simulink model "BatteryFarmTemplate"  (R2022b)
settings: Solver=VariableStepAuto  StartTime=0.0  StopTime=10.0  RelTol=1e-3  AbsTol=1e-3  EnableMultiTasking=on
libraries: ee_lib x242, sdl_lib x84, fl_lib x43
(part 5 of 5)

== system BatteryFarmTemplate/Battery Conex 1/Parallel Charge 6 ==
  Electrical Reference : fl_lib/Electrical/Electrical Elements/Electrical Reference
  Resistor 1 : ee_lib/Passive/Resistor  R=3200 Ohm  enable_R_tol=0  R_tol=5  tol_distribution=1  nSigma=4  enable_operating_limits=0  operating_limit_action=2  max_working_voltage=100 V  power_rating=1 W  enable_faults=0  fault_action=1  R_faulted=inf Ohm  enable_temporal_fault=0  t_fault=1 s  enable_behavioral_fault=0  max_permissible_current=1 A  t_fail_on_current=1 s  noise_mode=0  sample_time=1e-3 s  repeatability=1  auto_seed=4111000739  user_seed=0  Tdevice=25 degC  power_derating_T1=70 degC  power_derating_T2=155 degC  operating_temperature_range_vec=[-50, 150] degC  alpha=3.93e-3 1/K  Tmeas=25 degC  thermal_mass=100 J/K  temperature_specify=off  temperature_priority=High  temperature=298.15 K  temperature_nominal_specify=off  temperature_nominal_unit=K  temperature_nominal_value=1
  Resistor 2 : ee_lib/Passive/Resistor  R=450 Ohm  enable_R_tol=0  R_tol=5  tol_distribution=1  nSigma=4  enable_operating_limits=0  operating_limit_action=2  max_working_voltage=100 V  power_rating=1 W  enable_faults=0  fault_action=1  R_faulted=inf Ohm  enable_temporal_fault=0  t_fault=1 s  enable_behavioral_fault=0  max_permissible_current=1 A  t_fail_on_current=1 s  noise_mode=0  sample_time=1e-3 s  repeatability=1  auto_seed=2084672538  user_seed=0  Tdevice=25 degC  power_derating_T1=70 degC  power_derating_T2=155 degC  operating_temperature_range_vec=[-50, 150] degC  alpha=3.93e-3 1/K  Tmeas=25 degC  thermal_mass=100 J/K  temperature_specify=off  temperature_priority=High  temperature=298.15 K  temperature_nominal_specify=off  temperature_nominal_unit=K  temperature_nominal_value=1
  SPST Relay 1 : ee_lib/Switches & Breakers/Relays/SPST Relay  block_choices=ee.enum.controlport.ps  R_closed=0.01 Ohm  G_open=1e-8 1/Ohm  Threshold=0  exposemeasurement=ee.enum.exposemeasurement.hidden  V_rated=5 V  V_energize=75  V_deenergize=25  l_winding=0.08 H  r_winding=12.5 Ohm  g_winding=1e-9 1/Ohm  T_brk_C_S=0 s  T_mak_C_S=0 s  enable_faults=ee.enum.relays.enable.no  fault_action=ee.enum.relays.faultaction.none  fault_types=ee.enum.relays.faultTypes.winding  fault_condition_ps=ee.enum.relays.faultConditionSPSTps.csstuck  r_deg_closed_s=1e-9 Ohm  winding_tau_fault=1e-3 s  tau_fault=1e-3 s  enable_temporal_fault=ee.enum.relays.enable.no  t_fault_stick=1 s  t_fault_ComOpen=1 s  t_fault=1 s  enable_behavioral_fault=ee.enum.relays.enable.no  winding_max_permissible_voltage=inf V  n_fail_on_voltage=1  winding_max_permissible_current=inf A  max_permissible_current=inf A  t_fail_on_current=1 s
      settings: InternalSimscapePortConfiguration="{\"Bottom\":[],\"Left\":[{\"id\":\"PS\",\"label\":\"PS\",\"type\":\"input\"}],\"Right\":[{\"id\":\"S\",\"label\":\"S\",\"type\":\"foundation.electrical.electrical\"},{\"id\":\"COM\",\"label\":\"C\",\"type\":\"foundation.electrical.electrical\"}],\"Top\":[]}"
  SPST Relay 2 : ee_lib/Switches & Breakers/Relays/SPST Relay  block_choices=ee.enum.controlport.ps  R_closed=0.01 Ohm  G_open=1e-8 1/Ohm  Threshold=0  exposemeasurement=ee.enum.exposemeasurement.hidden  V_rated=5 V  V_energize=75  V_deenergize=25  l_winding=0.08 H  r_winding=12.5 Ohm  g_winding=1e-9 1/Ohm  T_brk_C_S=0 s  T_mak_C_S=0 s  enable_faults=ee.enum.relays.enable.no  fault_action=ee.enum.relays.faultaction.none  fault_types=ee.enum.relays.faultTypes.winding  fault_condition_ps=ee.enum.relays.faultConditionSPSTps.csstuck  r_deg_closed_s=1e-9 Ohm  winding_tau_fault=1e-3 s  tau_fault=1e-3 s  enable_temporal_fault=ee.enum.relays.enable.no  t_fault_stick=1 s  t_fault_ComOpen=1 s  t_fault=1 s  enable_behavioral_fault=ee.enum.relays.enable.no  winding_max_permissible_voltage=inf V  n_fail_on_voltage=1  winding_max_permissible_current=inf A  max_permissible_current=inf A  t_fail_on_current=1 s
      settings: InternalSimscapePortConfiguration="{\"Bottom\":[],\"Left\":[{\"id\":\"PS\",\"label\":\"PS\",\"type\":\"input\"}],\"Right\":[{\"id\":\"S\",\"label\":\"S\",\"type\":\"foundation.electrical.electrical\"},{\"id\":\"COM\",\"label\":\"C\",\"type\":\"foundation.electrical.electrical\"}],\"Top\":[]}"
  Charge Pos In : PMIOPort  Side=Left
  Charge Pos Out : PMIOPort  Port=2  Side=Left
  Energize Relay : PMIOPort  Port=3  Side=Left
  Charge Neg Out : PMIOPort  Port=4  Side=Right
  Charge Neg In : PMIOPort  Port=5  Side=Right
  connections:
  Electrical Reference/LConn1 -- Resistor 2/RConn1
  Resistor 2/LConn1 -- Resistor 1/LConn1 -- SPST Relay 1/RConn1
  SPST Relay 2/RConn2 -- Charge Neg Out/RConn1
  Charge Neg In/RConn1 -- SPST Relay 2/RConn1
  Resistor 1/RConn1 -- Charge Pos In/RConn1
  Charge Pos Out/RConn1 -- SPST Relay 1/RConn2
  SPST Relay 1/LConn1 -- Energize Relay/RConn1 -- SPST Relay 2/LConn1

== system BatteryFarmTemplate/Battery Conex 1/Parallel Charge 7 ==
  Electrical Reference : fl_lib/Electrical/Electrical Elements/Electrical Reference
  Resistor 1 : ee_lib/Passive/Resistor  R=3200 Ohm  enable_R_tol=0  R_tol=5  tol_distribution=1  nSigma=4  enable_operating_limits=0  operating_limit_action=2  max_working_voltage=100 V  power_rating=1 W  enable_faults=0  fault_action=1  R_faulted=inf Ohm  enable_temporal_fault=0  t_fault=1 s  enable_behavioral_fault=0  max_permissible_current=1 A  t_fail_on_current=1 s  noise_mode=0  sample_time=1e-3 s  repeatability=1  auto_seed=3437178441  user_seed=0  Tdevice=25 degC  power_derating_T1=70 degC  power_derating_T2=155 degC  operating_temperature_range_vec=[-50, 150] degC  alpha=3.93e-3 1/K  Tmeas=25 degC  thermal_mass=100 J/K  temperature_specify=off  temperature_priority=High  temperature=298.15 K  temperature_nominal_specify=off  temperature_nominal_unit=K  temperature_nominal_value=1
  Resistor 2 : ee_lib/Passive/Resistor  R=450 Ohm  enable_R_tol=0  R_tol=5  tol_distribution=1  nSigma=4  enable_operating_limits=0  operating_limit_action=2  max_working_voltage=100 V  power_rating=1 W  enable_faults=0  fault_action=1  R_faulted=inf Ohm  enable_temporal_fault=0  t_fault=1 s  enable_behavioral_fault=0  max_permissible_current=1 A  t_fail_on_current=1 s  noise_mode=0  sample_time=1e-3 s  repeatability=1  auto_seed=609397185  user_seed=0  Tdevice=25 degC  power_derating_T1=70 degC  power_derating_T2=155 degC  operating_temperature_range_vec=[-50, 150] degC  alpha=3.93e-3 1/K  Tmeas=25 degC  thermal_mass=100 J/K  temperature_specify=off  temperature_priority=High  temperature=298.15 K  temperature_nominal_specify=off  temperature_nominal_unit=K  temperature_nominal_value=1
  SPST Relay 1 : ee_lib/Switches & Breakers/Relays/SPST Relay  block_choices=ee.enum.controlport.ps  R_closed=0.01 Ohm  G_open=1e-8 1/Ohm  Threshold=0  exposemeasurement=ee.enum.exposemeasurement.hidden  V_rated=5 V  V_energize=75  V_deenergize=25  l_winding=0.08 H  r_winding=12.5 Ohm  g_winding=1e-9 1/Ohm  T_brk_C_S=0 s  T_mak_C_S=0 s  enable_faults=ee.enum.relays.enable.no  fault_action=ee.enum.relays.faultaction.none  fault_types=ee.enum.relays.faultTypes.winding  fault_condition_ps=ee.enum.relays.faultConditionSPSTps.csstuck  r_deg_closed_s=1e-9 Ohm  winding_tau_fault=1e-3 s  tau_fault=1e-3 s  enable_temporal_fault=ee.enum.relays.enable.no  t_fault_stick=1 s  t_fault_ComOpen=1 s  t_fault=1 s  enable_behavioral_fault=ee.enum.relays.enable.no  winding_max_permissible_voltage=inf V  n_fail_on_voltage=1  winding_max_permissible_current=inf A  max_permissible_current=inf A  t_fail_on_current=1 s
      settings: InternalSimscapePortConfiguration="{\"Bottom\":[],\"Left\":[{\"id\":\"PS\",\"label\":\"PS\",\"type\":\"input\"}],\"Right\":[{\"id\":\"S\",\"label\":\"S\",\"type\":\"foundation.electrical.electrical\"},{\"id\":\"COM\",\"label\":\"C\",\"type\":\"foundation.electrical.electrical\"}],\"Top\":[]}"
  SPST Relay 2 : ee_lib/Switches & Breakers/Relays/SPST Relay  block_choices=ee.enum.controlport.ps  R_closed=0.01 Ohm  G_open=1e-8 1/Ohm  Threshold=0  exposemeasurement=ee.enum.exposemeasurement.hidden  V_rated=5 V  V_energize=75  V_deenergize=25  l_winding=0.08 H  r_winding=12.5 Ohm  g_winding=1e-9 1/Ohm  T_brk_C_S=0 s  T_mak_C_S=0 s  enable_faults=ee.enum.relays.enable.no  fault_action=ee.enum.relays.faultaction.none  fault_types=ee.enum.relays.faultTypes.winding  fault_condition_ps=ee.enum.relays.faultConditionSPSTps.csstuck  r_deg_closed_s=1e-9 Ohm  winding_tau_fault=1e-3 s  tau_fault=1e-3 s  enable_temporal_fault=ee.enum.relays.enable.no  t_fault_stick=1 s  t_fault_ComOpen=1 s  t_fault=1 s  enable_behavioral_fault=ee.enum.relays.enable.no  winding_max_permissible_voltage=inf V  n_fail_on_voltage=1  winding_max_permissible_current=inf A  max_permissible_current=inf A  t_fail_on_current=1 s
      settings: InternalSimscapePortConfiguration="{\"Bottom\":[],\"Left\":[{\"id\":\"PS\",\"label\":\"PS\",\"type\":\"input\"}],\"Right\":[{\"id\":\"S\",\"label\":\"S\",\"type\":\"foundation.electrical.electrical\"},{\"id\":\"COM\",\"label\":\"C\",\"type\":\"foundation.electrical.electrical\"}],\"Top\":[]}"
  Charge Pos In : PMIOPort  Side=Left
  Charge Pos Out : PMIOPort  Port=2  Side=Left
  Energize Relay : PMIOPort  Port=3  Side=Left
  Charge Neg Out : PMIOPort  Port=4  Side=Right
  Charge Neg In : PMIOPort  Port=5  Side=Right
  connections:
  Electrical Reference/LConn1 -- Resistor 2/RConn1
  Resistor 2/LConn1 -- Resistor 1/LConn1 -- SPST Relay 1/RConn1
  SPST Relay 2/RConn2 -- Charge Neg Out/RConn1
  Charge Neg In/RConn1 -- SPST Relay 2/RConn1
  Resistor 1/RConn1 -- Charge Pos In/RConn1
  Charge Pos Out/RConn1 -- SPST Relay 1/RConn2
  SPST Relay 1/LConn1 -- Energize Relay/RConn1 -- SPST Relay 2/LConn1

== system BatteryFarmTemplate/Battery Conex 1/Parallel Charge 8 ==
  Electrical Reference : fl_lib/Electrical/Electrical Elements/Electrical Reference
  Resistor 1 : ee_lib/Passive/Resistor  R=3200 Ohm  enable_R_tol=0  R_tol=5  tol_distribution=1  nSigma=4  enable_operating_limits=0  operating_limit_action=2  max_working_voltage=100 V  power_rating=1 W  enable_faults=0  fault_action=1  R_faulted=inf Ohm  enable_temporal_fault=0  t_fault=1 s  enable_behavioral_fault=0  max_permissible_current=1 A  t_fail_on_current=1 s  noise_mode=0  sample_time=1e-3 s  repeatability=1  auto_seed=802611725  user_seed=0  Tdevice=25 degC  power_derating_T1=70 degC  power_derating_T2=155 degC  operating_temperature_range_vec=[-50, 150] degC  alpha=3.93e-3 1/K  Tmeas=25 degC  thermal_mass=100 J/K  temperature_specify=off  temperature_priority=High  temperature=298.15 K  temperature_nominal_specify=off  temperature_nominal_unit=K  temperature_nominal_value=1
  Resistor 2 : ee_lib/Passive/Resistor  R=450 Ohm  enable_R_tol=0  R_tol=5  tol_distribution=1  nSigma=4  enable_operating_limits=0  operating_limit_action=2  max_working_voltage=100 V  power_rating=1 W  enable_faults=0  fault_action=1  R_faulted=inf Ohm  enable_temporal_fault=0  t_fault=1 s  enable_behavioral_fault=0  max_permissible_current=1 A  t_fail_on_current=1 s  noise_mode=0  sample_time=1e-3 s  repeatability=1  auto_seed=2103522063  user_seed=0  Tdevice=25 degC  power_derating_T1=70 degC  power_derating_T2=155 degC  operating_temperature_range_vec=[-50, 150] degC  alpha=3.93e-3 1/K  Tmeas=25 degC  thermal_mass=100 J/K  temperature_specify=off  temperature_priority=High  temperature=298.15 K  temperature_nominal_specify=off  temperature_nominal_unit=K  temperature_nominal_value=1
  SPST Relay 1 : ee_lib/Switches & Breakers/Relays/SPST Relay  block_choices=ee.enum.controlport.ps  R_closed=0.01 Ohm  G_open=1e-8 1/Ohm  Threshold=0  exposemeasurement=ee.enum.exposemeasurement.hidden  V_rated=5 V  V_energize=75  V_deenergize=25  l_winding=0.08 H  r_winding=12.5 Ohm  g_winding=1e-9 1/Ohm  T_brk_C_S=0 s  T_mak_C_S=0 s  enable_faults=ee.enum.relays.enable.no  fault_action=ee.enum.relays.faultaction.none  fault_types=ee.enum.relays.faultTypes.winding  fault_condition_ps=ee.enum.relays.faultConditionSPSTps.csstuck  r_deg_closed_s=1e-9 Ohm  winding_tau_fault=1e-3 s  tau_fault=1e-3 s  enable_temporal_fault=ee.enum.relays.enable.no  t_fault_stick=1 s  t_fault_ComOpen=1 s  t_fault=1 s  enable_behavioral_fault=ee.enum.relays.enable.no  winding_max_permissible_voltage=inf V  n_fail_on_voltage=1  winding_max_permissible_current=inf A  max_permissible_current=inf A  t_fail_on_current=1 s
      settings: InternalSimscapePortConfiguration="{\"Bottom\":[],\"Left\":[{\"id\":\"PS\",\"label\":\"PS\",\"type\":\"input\"}],\"Right\":[{\"id\":\"S\",\"label\":\"S\",\"type\":\"foundation.electrical.electrical\"},{\"id\":\"COM\",\"label\":\"C\",\"type\":\"foundation.electrical.electrical\"}],\"Top\":[]}"
  SPST Relay 2 : ee_lib/Switches & Breakers/Relays/SPST Relay  block_choices=ee.enum.controlport.ps  R_closed=0.01 Ohm  G_open=1e-8 1/Ohm  Threshold=0  exposemeasurement=ee.enum.exposemeasurement.hidden  V_rated=5 V  V_energize=75  V_deenergize=25  l_winding=0.08 H  r_winding=12.5 Ohm  g_winding=1e-9 1/Ohm  T_brk_C_S=0 s  T_mak_C_S=0 s  enable_faults=ee.enum.relays.enable.no  fault_action=ee.enum.relays.faultaction.none  fault_types=ee.enum.relays.faultTypes.winding  fault_condition_ps=ee.enum.relays.faultConditionSPSTps.csstuck  r_deg_closed_s=1e-9 Ohm  winding_tau_fault=1e-3 s  tau_fault=1e-3 s  enable_temporal_fault=ee.enum.relays.enable.no  t_fault_stick=1 s  t_fault_ComOpen=1 s  t_fault=1 s  enable_behavioral_fault=ee.enum.relays.enable.no  winding_max_permissible_voltage=inf V  n_fail_on_voltage=1  winding_max_permissible_current=inf A  max_permissible_current=inf A  t_fail_on_current=1 s
      settings: InternalSimscapePortConfiguration="{\"Bottom\":[],\"Left\":[{\"id\":\"PS\",\"label\":\"PS\",\"type\":\"input\"}],\"Right\":[{\"id\":\"S\",\"label\":\"S\",\"type\":\"foundation.electrical.electrical\"},{\"id\":\"COM\",\"label\":\"C\",\"type\":\"foundation.electrical.electrical\"}],\"Top\":[]}"
  Charge Pos In : PMIOPort  Side=Left
  Charge Pos Out : PMIOPort  Port=2  Side=Left
  Energize Relay : PMIOPort  Port=3  Side=Left
  Charge Neg Out : PMIOPort  Port=4  Side=Right
  Charge Neg In : PMIOPort  Port=5  Side=Right
  connections:
  Electrical Reference/LConn1 -- Resistor 2/RConn1
  Resistor 2/LConn1 -- Resistor 1/LConn1 -- SPST Relay 1/RConn1
  SPST Relay 2/RConn2 -- Charge Neg Out/RConn1
  Charge Neg In/RConn1 -- SPST Relay 2/RConn1
  Resistor 1/RConn1 -- Charge Pos In/RConn1
  Charge Pos Out/RConn1 -- SPST Relay 1/RConn2
  SPST Relay 1/LConn1 -- Energize Relay/RConn1 -- SPST Relay 2/LConn1

== system BatteryFarmTemplate/Battery Conex 1/Parallel Charge 9 ==
  Electrical Reference : fl_lib/Electrical/Electrical Elements/Electrical Reference
  Resistor 1 : ee_lib/Passive/Resistor  R=3200 Ohm  enable_R_tol=0  R_tol=5  tol_distribution=1  nSigma=4  enable_operating_limits=0  operating_limit_action=2  max_working_voltage=100 V  power_rating=1 W  enable_faults=0  fault_action=1  R_faulted=inf Ohm  enable_temporal_fault=0  t_fault=1 s  enable_behavioral_fault=0  max_permissible_current=1 A  t_fail_on_current=1 s  noise_mode=0  sample_time=1e-3 s  repeatability=1  auto_seed=1913778160  user_seed=0  Tdevice=25 degC  power_derating_T1=70 degC  power_derating_T2=155 degC  operating_temperature_range_vec=[-50, 150] degC  alpha=3.93e-3 1/K  Tmeas=25 degC  thermal_mass=100 J/K  temperature_specify=off  temperature_priority=High  temperature=298.15 K  temperature_nominal_specify=off  temperature_nominal_unit=K  temperature_nominal_value=1
  Resistor 2 : ee_lib/Passive/Resistor  R=450 Ohm  enable_R_tol=0  R_tol=5  tol_distribution=1  nSigma=4  enable_operating_limits=0  operating_limit_action=2  max_working_voltage=100 V  power_rating=1 W  enable_faults=0  fault_action=1  R_faulted=inf Ohm  enable_temporal_fault=0  t_fault=1 s  enable_behavioral_fault=0  max_permissible_current=1 A  t_fail_on_current=1 s  noise_mode=0  sample_time=1e-3 s  repeatability=1  auto_seed=2775893241  user_seed=0  Tdevice=25 degC  power_derating_T1=70 degC  power_derating_T2=155 degC  operating_temperature_range_vec=[-50, 150] degC  alpha=3.93e-3 1/K  Tmeas=25 degC  thermal_mass=100 J/K  temperature_specify=off  temperature_priority=High  temperature=298.15 K  temperature_nominal_specify=off  temperature_nominal_unit=K  temperature_nominal_value=1
  SPST Relay 1 : ee_lib/Switches & Breakers/Relays/SPST Relay  block_choices=ee.enum.controlport.ps  R_closed=0.01 Ohm  G_open=1e-8 1/Ohm  Threshold=0  exposemeasurement=ee.enum.exposemeasurement.hidden  V_rated=5 V  V_energize=75  V_deenergize=25  l_winding=0.08 H  r_winding=12.5 Ohm  g_winding=1e-9 1/Ohm  T_brk_C_S=0 s  T_mak_C_S=0 s  enable_faults=ee.enum.relays.enable.no  fault_action=ee.enum.relays.faultaction.none  fault_types=ee.enum.relays.faultTypes.winding  fault_condition_ps=ee.enum.relays.faultConditionSPSTps.csstuck  r_deg_closed_s=1e-9 Ohm  winding_tau_fault=1e-3 s  tau_fault=1e-3 s  enable_temporal_fault=ee.enum.relays.enable.no  t_fault_stick=1 s  t_fault_ComOpen=1 s  t_fault=1 s  enable_behavioral_fault=ee.enum.relays.enable.no  winding_max_permissible_voltage=inf V  n_fail_on_voltage=1  winding_max_permissible_current=inf A  max_permissible_current=inf A  t_fail_on_current=1 s
      settings: InternalSimscapePortConfiguration="{\"Bottom\":[],\"Left\":[{\"id\":\"PS\",\"label\":\"PS\",\"type\":\"input\"}],\"Right\":[{\"id\":\"S\",\"label\":\"S\",\"type\":\"foundation.electrical.electrical\"},{\"id\":\"COM\",\"label\":\"C\",\"type\":\"foundation.electrical.electrical\"}],\"Top\":[]}"
  SPST Relay 2 : ee_lib/Switches & Breakers/Relays/SPST Relay  block_choices=ee.enum.controlport.ps  R_closed=0.01 Ohm  G_open=1e-8 1/Ohm  Threshold=0  exposemeasurement=ee.enum.exposemeasurement.hidden  V_rated=5 V  V_energize=75  V_deenergize=25  l_winding=0.08 H  r_winding=12.5 Ohm  g_winding=1e-9 1/Ohm  T_brk_C_S=0 s  T_mak_C_S=0 s  enable_faults=ee.enum.relays.enable.no  fault_action=ee.enum.relays.faultaction.none  fault_types=ee.enum.relays.faultTypes.winding  fault_condition_ps=ee.enum.relays.faultConditionSPSTps.csstuck  r_deg_closed_s=1e-9 Ohm  winding_tau_fault=1e-3 s  tau_fault=1e-3 s  enable_temporal_fault=ee.enum.relays.enable.no  t_fault_stick=1 s  t_fault_ComOpen=1 s  t_fault=1 s  enable_behavioral_fault=ee.enum.relays.enable.no  winding_max_permissible_voltage=inf V  n_fail_on_voltage=1  winding_max_permissible_current=inf A  max_permissible_current=inf A  t_fail_on_current=1 s
      settings: InternalSimscapePortConfiguration="{\"Bottom\":[],\"Left\":[{\"id\":\"PS\",\"label\":\"PS\",\"type\":\"input\"}],\"Right\":[{\"id\":\"S\",\"label\":\"S\",\"type\":\"foundation.electrical.electrical\"},{\"id\":\"COM\",\"label\":\"C\",\"type\":\"foundation.electrical.electrical\"}],\"Top\":[]}"
  Charge Pos In : PMIOPort  Side=Left
  Charge Pos Out : PMIOPort  Port=2  Side=Left
  Energize Relay : PMIOPort  Port=3  Side=Left
  Charge Neg Out : PMIOPort  Port=4  Side=Right
  Charge Neg In : PMIOPort  Port=5  Side=Right
  connections:
  Electrical Reference/LConn1 -- Resistor 2/RConn1
  Resistor 2/LConn1 -- Resistor 1/LConn1 -- SPST Relay 1/RConn1
  SPST Relay 2/RConn2 -- Charge Neg Out/RConn1
  Charge Neg In/RConn1 -- SPST Relay 2/RConn1
  Resistor 1/RConn1 -- Charge Pos In/RConn1
  Charge Pos Out/RConn1 -- SPST Relay 1/RConn2
  SPST Relay 1/LConn1 -- Energize Relay/RConn1 -- SPST Relay 2/LConn1

== system BatteryFarmTemplate/Battery Conex 1/Parallel Relay Control ==
  Parallel 1 : PMIOPort  Side=Right
  Parallel 2 : PMIOPort  Port=2  Side=Right
  Parallel 3 : PMIOPort  Port=3  Side=Right
  Parallel 4 : PMIOPort  Port=4  Side=Right
  Parallel 5 : PMIOPort  Port=5  Side=Right
  Parallel 6 : PMIOPort  Port=6  Side=Right
  Parallel 7 : PMIOPort  Port=7  Side=Right
  Parallel 8 : PMIOPort  Port=8  Side=Right
  Parallel 9 : PMIOPort  Port=9  Side=Right
  Parallel 10 : PMIOPort  Port=10  Side=Right
  Parallel 11 : PMIOPort  Port=11  Side=Right
  Parallel 12 : PMIOPort  Port=12  Side=Right
  Parallel 13 : PMIOPort  Port=13  Side=Right
  Parallel 14 : PMIOPort  Port=14  Side=Right

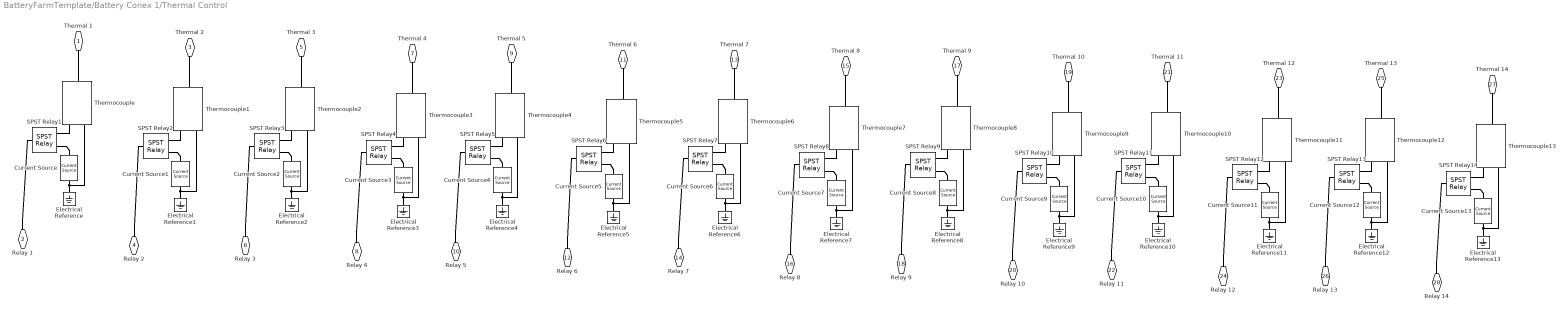
== system BatteryFarmTemplate/Battery Conex 1/Thermal Control ==
  Current Source : ee_lib/Sources/Current Source  dc_current=44 A  ac_current=0 A  ac_shift=0 rad  ac_frequency=50 Hz  noise_mode=ee.enum.sources.noise.Disabled  PSD=0 A^2/Hz  sample_time=1e-3 s  repeatability=ee.enum.sources.repeatability.NotRepeatable  user_seed=0  auto_seed=3890346746  i_specify=off  i_priority=None  i=0 A  i_nominal_specify=off  i_nominal_unit=A  i_nominal_value=1  v_specify=off  v_priority=None  v=0 V  v_nominal_specify=off  v_nominal_unit=V  v_nominal_value=1
  Current Source1 : ee_lib/Sources/Current Source  dc_current=44 A  ac_current=0 A  ac_shift=0 rad  ac_frequency=50 Hz  noise_mode=ee.enum.sources.noise.Disabled  PSD=0 A^2/Hz  sample_time=1e-3 s  repeatability=ee.enum.sources.repeatability.NotRepeatable  user_seed=0  auto_seed=609397185  i_specify=off  i_priority=None  i=0 A  i_nominal_specify=off  i_nominal_unit=A  i_nominal_value=1  v_specify=off  v_priority=None  v=0 V  v_nominal_specify=off  v_nominal_unit=V  v_nominal_value=1
  Current Source10 : ee_lib/Sources/Current Source  dc_current=44 A  ac_current=0 A  ac_shift=0 rad  ac_frequency=50 Hz  noise_mode=ee.enum.sources.noise.Disabled  PSD=0 A^2/Hz  sample_time=1e-3 s  repeatability=ee.enum.sources.repeatability.NotRepeatable  user_seed=0  auto_seed=2816384857  i_specify=off  i_priority=None  i=0 A  i_nominal_specify=off  i_nominal_unit=A  i_nominal_value=1  v_specify=off  v_priority=None  v=0 V  v_nominal_specify=off  v_nominal_unit=V  v_nominal_value=1
  Current Source11 : ee_lib/Sources/Current Source  dc_current=44 A  ac_current=0 A  ac_shift=0 rad  ac_frequency=50 Hz  noise_mode=ee.enum.sources.noise.Disabled  PSD=0 A^2/Hz  sample_time=1e-3 s  repeatability=ee.enum.sources.repeatability.NotRepeatable  user_seed=0  auto_seed=153380492  i_specify=off  i_priority=None  i=0 A  i_nominal_specify=off  i_nominal_unit=A  i_nominal_value=1  v_specify=off  v_priority=None  v=0 V  v_nominal_specify=off  v_nominal_unit=V  v_nominal_value=1
  Current Source12 : ee_lib/Sources/Current Source  dc_current=44 A  ac_current=0 A  ac_shift=0 rad  ac_frequency=50 Hz  noise_mode=ee.enum.sources.noise.Disabled  PSD=0 A^2/Hz  sample_time=1e-3 s  repeatability=ee.enum.sources.repeatability.NotRepeatable  user_seed=0  auto_seed=3191729647  i_specify=off  i_priority=None  i=0 A  i_nominal_specify=off  i_nominal_unit=A  i_nominal_value=1  v_specify=off  v_priority=None  v=0 V  v_nominal_specify=off  v_nominal_unit=V  v_nominal_value=1
  Current Source13 : ee_lib/Sources/Current Source  dc_current=44 A  ac_current=0 A  ac_shift=0 rad  ac_frequency=50 Hz  noise_mode=ee.enum.sources.noise.Disabled  PSD=0 A^2/Hz  sample_time=1e-3 s  repeatability=ee.enum.sources.repeatability.NotRepeatable  user_seed=0  auto_seed=1684602222  i_specify=off  i_priority=None  i=0 A  i_nominal_specify=off  i_nominal_unit=A  i_nominal_value=1  v_specify=off  v_priority=None  v=0 V  v_nominal_specify=off  v_nominal_unit=V  v_nominal_value=1
  Current Source2 : ee_lib/Sources/Current Source  dc_current=44 A  ac_current=0 A  ac_shift=0 rad  ac_frequency=50 Hz  noise_mode=ee.enum.sources.noise.Disabled  PSD=0 A^2/Hz  sample_time=1e-3 s  repeatability=ee.enum.sources.repeatability.NotRepeatable  user_seed=0  auto_seed=1811450916  i_specify=off  i_priority=None  i=0 A  i_nominal_specify=off  i_nominal_unit=A  i_nominal_value=1  v_specify=off  v_priority=None  v=0 V  v_nominal_specify=off  v_nominal_unit=V  v_nominal_value=1
  Current Source3 : ee_lib/Sources/Current Source  dc_current=44 A  ac_current=0 A  ac_shift=0 rad  ac_frequency=50 Hz  noise_mode=ee.enum.sources.noise.Disabled  PSD=0 A^2/Hz  sample_time=1e-3 s  repeatability=ee.enum.sources.repeatability.NotRepeatable  user_seed=0  auto_seed=3933054132  i_specify=off  i_priority=None  i=0 A  i_nominal_specify=off  i_nominal_unit=A  i_nominal_value=1  v_specify=off  v_priority=None  v=0 V  v_nominal_specify=off  v_nominal_unit=V  v_nominal_value=1
  Current Source4 : ee_lib/Sources/Current Source  dc_current=44 A  ac_current=0 A  ac_shift=0 rad  ac_frequency=50 Hz  noise_mode=ee.enum.sources.noise.Disabled  PSD=0 A^2/Hz  sample_time=1e-3 s  repeatability=ee.enum.sources.repeatability.NotRepeatable  user_seed=0  auto_seed=3402504572  i_specify=off  i_priority=None  i=0 A  i_nominal_specify=off  i_nominal_unit=A  i_nominal_value=1  v_specify=off  v_priority=None  v=0 V  v_nominal_specify=off  v_nominal_unit=V  v_nominal_value=1
  Current Source5 : ee_lib/Sources/Current Source  dc_current=44 A  ac_current=0 A  ac_shift=0 rad  ac_frequency=50 Hz  noise_mode=ee.enum.sources.noise.Disabled  PSD=0 A^2/Hz  sample_time=1e-3 s  repeatability=ee.enum.sources.repeatability.NotRepeatable  user_seed=0  auto_seed=4120988592  i_specify=off  i_priority=None  i=0 A  i_nominal_specify=off  i_nominal_unit=A  i_nominal_value=1  v_specify=off  v_priority=None  v=0 V  v_nominal_specify=off  v_nominal_unit=V  v_nominal_value=1
  Current Source6 : ee_lib/Sources/Current Source  dc_current=44 A  ac_current=0 A  ac_shift=0 rad  ac_frequency=50 Hz  noise_mode=ee.enum.sources.noise.Disabled  PSD=0 A^2/Hz  sample_time=1e-3 s  repeatability=ee.enum.sources.repeatability.NotRepeatable  user_seed=0  auto_seed=3646982598  i_specify=off  i_priority=None  i=0 A  i_nominal_specify=off  i_nominal_unit=A  i_nominal_value=1  v_specify=off  v_priority=None  v=0 V  v_nominal_specify=off  v_nominal_unit=V  v_nominal_value=1
  Current Source7 : ee_lib/Sources/Current Source  dc_current=44 A  ac_current=0 A  ac_shift=0 rad  ac_frequency=50 Hz  noise_mode=ee.enum.sources.noise.Disabled  PSD=0 A^2/Hz  sample_time=1e-3 s  repeatability=ee.enum.sources.repeatability.NotRepeatable  user_seed=0  auto_seed=4011470453  i_specify=off  i_priority=None  i=0 A  i_nominal_specify=off  i_nominal_unit=A  i_nominal_value=1  v_specify=off  v_priority=None  v=0 V  v_nominal_specify=off  v_nominal_unit=V  v_nominal_value=1
  Current Source8 : ee_lib/Sources/Current Source  dc_current=44 A  ac_current=0 A  ac_shift=0 rad  ac_frequency=50 Hz  noise_mode=ee.enum.sources.noise.Disabled  PSD=0 A^2/Hz  sample_time=1e-3 s  repeatability=ee.enum.sources.repeatability.NotRepeatable  user_seed=0  auto_seed=2915145293  i_specify=off  i_priority=None  i=0 A  i_nominal_specify=off  i_nominal_unit=A  i_nominal_value=1  v_specify=off  v_priority=None  v=0 V  v_nominal_specify=off  v_nominal_unit=V  v_nominal_value=1
  Current Source9 : ee_lib/Sources/Current Source  dc_current=44 A  ac_current=0 A  ac_shift=0 rad  ac_frequency=50 Hz  noise_mode=ee.enum.sources.noise.Disabled  PSD=0 A^2/Hz  sample_time=1e-3 s  repeatability=ee.enum.sources.repeatability.NotRepeatable  user_seed=0  auto_seed=3254469079  i_specify=off  i_priority=None  i=0 A  i_nominal_specify=off  i_nominal_unit=A  i_nominal_value=1  v_specify=off  v_priority=None  v=0 V  v_nominal_specify=off  v_nominal_unit=V  v_nominal_value=1
  Electrical Reference{,1..13} (14 alike) : fl_lib/Electrical/Electrical Elements/Electrical Reference
  SPST Relay{1..14} (14 alike) : ee_lib/Switches & Breakers/Relays/SPST Relay  block_choices=ee.enum.controlport.ps  R_closed=0.01 Ohm  G_open=1e-8 1/Ohm  Threshold=0  exposemeasurement=ee.enum.exposemeasurement.hidden  V_rated=5 V  V_energize=75  V_deenergize=25  l_winding=0.08 H  r_winding=12.5 Ohm  g_winding=1e-9 1/Ohm  T_brk_C_S=0 s  T_mak_C_S=0 s  enable_faults=ee.enum.relays.enable.no  fault_action=ee.enum.relays.faultaction.none  fault_types=ee.enum.relays.faultTypes.winding  fault_condition_ps=ee.enum.relays.faultConditionSPSTps.csstuck  r_deg_closed_s=1e-9 Ohm  winding_tau_fault=1e-3 s  tau_fault=1e-3 s  enable_temporal_fault=ee.enum.relays.enable.no  t_fault_stick=1 s  t_fault_ComOpen=1 s  t_fault=1 s  enable_behavioral_fault=ee.enum.relays.enable.no  winding_max_permissible_voltage=inf V  n_fail_on_voltage=1  winding_max_permissible_current=inf A  max_permissible_current=inf A  t_fail_on_current=1 s
      settings: InternalSimscapePortConfiguration="{\"Bottom\":[],\"Left\":[{\"id\":\"PS\",\"label\":\"PS\",\"type\":\"input\"}],\"Right\":[{\"id\":\"S\",\"label\":\"S\",\"type\":\"foundation.electrical.electrical\"},{\"id\":\"COM\",\"label\":\"C\",\"type\":\"foundation.electrical.electrical\"}],\"Top\":[]}"
  Thermocouple{,1..13} (14 alike) : ee_lib/Sensors & Transducers/Thermocouple  thermocouple_type=1  Cvec=[0, 0, 0, 0, 0, 0, 0, 0, 0]  Avec=[0, 0, 0]  T0=0 degC  tc=1 s  K_d=1e-3 W/K  init_temp=25 degC
      settings: InternalSimscapePortConfiguration="{\"Bottom\":[],\"Left\":[{\"id\":\"p\",\"label\":\"+\",\"type\":\"foundation.electrical.electrical\"},{\"id\":\"n\",\"label\":\"-\",\"type\":\"foundation.electrical.electrical\"}],\"Right\":[{\"id\":\"A\",\"label\":\"A\",\"type\":\"foundation.thermal.thermal\"}],\"Top\":[]}"
  Thermal 1 : PMIOPort  Side=Left
  Relay 1 : PMIOPort  Port=2  Side=Right
  Thermal 2 : PMIOPort  Port=3  Side=Left
  Relay 2 : PMIOPort  Port=4  Side=Right
  Thermal 3 : PMIOPort  Port=5  Side=Left
  Relay 3 : PMIOPort  Port=6  Side=Right
  Thermal 4 : PMIOPort  Port=7  Side=Left
  Relay 4 : PMIOPort  Port=8  Side=Right
  Thermal 5 : PMIOPort  Port=9  Side=Left
  Relay 5 : PMIOPort  Port=10  Side=Right
  Thermal 6 : PMIOPort  Port=11  Side=Left
  Relay 6 : PMIOPort  Port=12  Side=Right
  Thermal 7 : PMIOPort  Port=13  Side=Left
  Relay 7 : PMIOPort  Port=14  Side=Right
  Thermal 8 : PMIOPort  Port=15  Side=Left
  Relay 8 : PMIOPort  Port=16  Side=Right
  Thermal 9 : PMIOPort  Port=17  Side=Left
  Relay 9 : PMIOPort  Port=18  Side=Right
  Thermal 10 : PMIOPort  Port=19  Side=Left
  Relay 10 : PMIOPort  Port=20  Side=Right
  Thermal 11 : PMIOPort  Port=21  Side=Left
  Relay 11 : PMIOPort  Port=22  Side=Right
  Thermal 12 : PMIOPort  Port=23  Side=Left
  Relay 12 : PMIOPort  Port=24  Side=Right
  Thermal 13 : PMIOPort  Port=25  Side=Left
  Relay 13 : PMIOPort  Port=26  Side=Right
  Thermal 14 : PMIOPort  Port=27  Side=Left
  Relay 14 : PMIOPort  Port=28  Side=Right
  connections:
  SPST Relay1/RConn1 -- Current Source/LConn1
  Electrical Reference/LConn1 -- Thermocouple/LConn2 -- Current Source/RConn1
  Relay 1/RConn1 -- SPST Relay1/LConn1
  Thermocouple/LConn1 -- SPST Relay1/RConn2
  Thermal 1/RConn1 -- Thermocouple/RConn1
  Electrical Reference1/LConn1 -- Thermocouple1/LConn2 -- Current Source1/RConn1
  Relay 2/RConn1 -- SPST Relay2/LConn1
  Thermal 2/RConn1 -- Thermocouple1/RConn1
  Thermocouple1/LConn1 -- SPST Relay2/RConn2
  SPST Relay2/RConn1 -- Current Source1/LConn1
  Electrical Reference3/LConn1 -- Thermocouple3/LConn2 -- Current Source3/RConn1
  Electrical Reference2/LConn1 -- Thermocouple2/LConn2 -- Current Source2/RConn1
  Thermal 4/RConn1 -- Thermocouple3/RConn1
  Relay 4/RConn1 -- SPST Relay4/LConn1
  SPST Relay4/RConn1 -- Current Source3/LConn1
  Thermocouple3/LConn1 -- SPST Relay4/RConn2
  Relay 3/RConn1 -- SPST Relay3/LConn1
  Thermal 3/RConn1 -- Thermocouple2/RConn1
  Thermocouple2/LConn1 -- SPST Relay3/RConn2
  SPST Relay3/RConn1 -- Current Source2/LConn1
  Electrical Reference5/LConn1 -- Thermocouple5/LConn2 -- Current Source5/RConn1
  Electrical Reference4/LConn1 -- Thermocouple4/LConn2 -- Current Source4/RConn1
  Thermal 6/RConn1 -- Thermocouple5/RConn1
  Relay 6/RConn1 -- SPST Relay6/LConn1
  SPST Relay6/RConn1 -- Current Source5/LConn1
  Thermocouple5/LConn1 -- SPST Relay6/RConn2
  Relay 5/RConn1 -- SPST Relay5/LConn1
  Thermal 5/RConn1 -- Thermocouple4/RConn1
  Thermocouple4/LConn1 -- SPST Relay5/RConn2
  SPST Relay5/RConn1 -- Current Source4/LConn1
  Electrical Reference9/LConn1 -- Thermocouple9/LConn2 -- Current Source9/RConn1
  Electrical Reference7/LConn1 -- Thermocouple7/LConn2 -- Current Source7/RConn1
  Electrical Reference11/LConn1 -- Thermocouple11/LConn2 -- Current Source11/RConn1
  Electrical Reference6/LConn1 -- Thermocouple6/LConn2 -- Current Source6/RConn1
  Electrical Reference10/LConn1 -- Thermocouple10/LConn2 -- Current Source10/RConn1
  Electrical Reference8/LConn1 -- Thermocouple8/LConn2 -- Current Source8/RConn1
  SPST Relay12/RConn1 -- Current Source11/LConn1
  Thermal 8/RConn1 -- Thermocouple7/RConn1
  Thermocouple6/LConn1 -- SPST Relay7/RConn2
  SPST Relay8/RConn1 -- Current Source7/LConn1
  Thermal 7/RConn1 -- Thermocouple6/RConn1
  Thermocouple7/LConn1 -- SPST Relay8/RConn2
  Relay 9/RConn1 -- SPST Relay9/LConn1
  Thermal 9/RConn1 -- Thermocouple8/RConn1
  SPST Relay9/RConn1 -- Current Source8/LConn1
  Relay 11/RConn1 -- SPST Relay11/LConn1
  Thermal 10/RConn1 -- Thermocouple9/RConn1
  Thermocouple9/LConn1 -- SPST Relay10/RConn2
  SPST Relay10/RConn1 -- Current Source9/LConn1
  SPST Relay7/RConn1 -- Current Source6/LConn1
  Thermal 11/RConn1 -- Thermocouple10/RConn1
  Thermocouple10/LConn1 -- SPST Relay11/RConn2
  SPST Relay11/RConn1 -- Current Source10/LConn1
  Thermocouple11/LConn1 -- SPST Relay12/RConn2
  Relay 8/RConn1 -- SPST Relay8/LConn1
  Thermocouple8/LConn1 -- SPST Relay9/RConn2
  Relay 10/RConn1 -- SPST Relay10/LConn1
  Relay 7/RConn1 -- SPST Relay7/LConn1
  Thermal 12/RConn1 -- Thermocouple11/RConn1
  Relay 12/RConn1 -- SPST Relay12/LConn1
  Electrical Reference13/LConn1 -- Thermocouple13/LConn2 -- Current Source13/RConn1
  Electrical Reference12/LConn1 -- Thermocouple12/LConn2 -- Current Source12/RConn1
  Relay 14/RConn1 -- SPST Relay14/LConn1
  Thermal 14/RConn1 -- Thermocouple13/RConn1
  Relay 13/RConn1 -- SPST Relay13/LConn1
  Thermocouple13/LConn1 -- SPST Relay14/RConn2
  Thermal 13/RConn1 -- Thermocouple12/RConn1
  SPST Relay14/RConn1 -- Current Source13/LConn1
  SPST Relay13/RConn1 -- Current Source12/LConn1
  Thermocouple12/LConn1 -- SPST Relay13/RConn2
